simulink model "adc083000"  (R2013b)
settings: Solver=FixedStepDiscrete  SolverMode=SingleTasking  StartTime=0.0  StopTime=10.0  RelTol=1e-3
libraries: xbsIndex_r4 x18, xps_library x13, dspsigops x8
settings Model: Creator=franco  LastModifiedBy=root
settings DebuggingCC: SolverPrmCheckMsg=none  StateNameClashWarn=warning

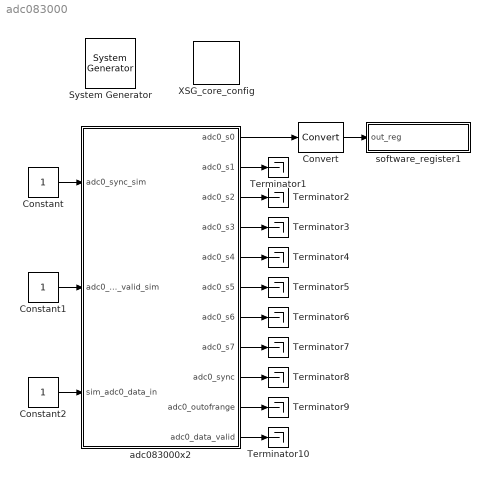
== system adc083000 ==
  " System Generator" : xbsIndex_r4/ System Generator  Tag=genX  xilinxfamily=virtex5  part=xc5vsx95t  speed=-1  package=ff1136  synthesis_tool=XST  clock_wrapper=Clock Enables  directory=./adc083000/sysgen  proj_type=Project Navigator  Synth_file=XST Defaults  Impl_file=ISE Defaults  testbench=off  simulink_period=1  sysclk_period=8.3333  dcm_input_clock_period=100  incr_netlist=off  trim_vbits=Everywhere in SubSystem  dbl_ovrd=According to Block Masks  core_generation=According to Block Masks  run_coregen=off  deprecated_control=off  eval_field=0  block_type=sysgen
  Constant : Constant
  Constant1 : Constant
  Constant2 : Constant
  Convert : xbsIndex_r4/Convert  gui_display_data_type=Fixed-point  arith_type=Unsigned  n_bits=32  bin_pt=0  float_type=Single  exp_bits=8  fraction_bits=24  quantization=Truncate  overflow=Wrap  en=off  latency=0  dbl_ovrd=off  pipeline=off  block_type=convert
  Terminator{1..10} (10 alike) : Terminator
  XSG_core_config : xps_library/XSG_core_config  Tag=xps:xsg  hw_sys=ROACH:sx95t  clk_src=adc0_clk  ROACH_clk_src=adc0_clk  ROACH2_clk_src=sys_clk  MKDIG_clk_src=sys_clk  clk_rate=120  sample_period=1  synthesis_tool=XST
  adc083000x2 : Subsystem  Tag=xps:adc083000x2  AncestorBlock=xps_library/adc083000x2  mask(adc_083000x2){use_adc0=on, use_adc1=off, demux_adc=off, clock_sync=off, verbose=off, using_ctrl=on, adc_clk_rate=480, sample_period=1, bit_width=8}
      mask prompts: use_adc0 "Use ZD0K0?"; use_adc1 "Use ZDOK1?"; demux_adc "Demux ADCs by 2?"; clock_sync "Interleave 2 ADC boards?"; verbose "Verbose Block Creation?"; using_ctrl "Add ports for control registers?"; adc_clk_rate "ADC clock rate (MHz)"; sample_period "Sample Period"; bit_width "Output Bit Width"
      mask help:
      | The ADC block converts analog inputs to digital outputs.
      | Every clock cycle, the inputs are sampled and digitized to
      | 8 bit binary point numbers in the range of [-1, 1).
      |
      | Online block-specific documentation: http://casper.berkeley.edu/wiki/Adc083000
      mask init:
      | adc083000_mask;
      mask Help: eval('xlWeb([getenv(''MLIB_ROOT''), ''\doc\html\sys_adc\sys_adc.html''])')
  software_register1 : Subsystem  Tag=xps:sw_reg  AncestorBlock=xps_library/software_register  mask(swreg){io_dir=To Processor, io_delay=0, sample_period=1, names=reg, bitwidths=32, bin_pts=0, arith_types=0, sim_port=off, show_format=on}
      mask prompts: io_dir "I/O direction"; io_delay "I/O delay"; sample_period "Sample period"; names "Bitfield names [msb...lsb]"; bitwidths "Bitfield widths"; bin_pts "Bitfield binary pts"; arith_types "Bitfield types, ufix=0, fix=1, bool=2"; sim_port "Provide sim input/output?"; show_format "Print format string?"
      mask help: A 32-bit software-accessible register. Can be divided into bitfields of varying widths and types using the fields in the block mask.
      mask init:
      | try
      |     swreg_init(gcb)
      | catch ex
      |     disp(sprintf('%s: %s', gcb, ex.message))
      |     errordlg(ex.message)
      | end
      settings: AttributesFormatString=1output:uf32.0 = 32 bits
      mask TypeOptions io_dir: To Processor | From Processor
      mask Callback io_dir:
      | mask_enables = get_param(gcb, 'MaskEnables');
      | mask_names = get_param(gcb, 'MaskNames');
      | if strcmp(get_param(gcb, 'io_dir'), 'To Processor'),
      |     mask_enables{ismember(mask_names, 'sample_period')} = 'off';
      | else
      |     mask_enables{ismember(mask_names, 'sample_period')} = 'on';
      | end
      | set_param(gcb, 'MaskEnables', mask_enables);
  wires:
  adc083000x2/1(adc0_s0) -> Convert/1
  adc083000x2/2(adc0_s1) -> Terminator1/1
  adc083000x2/3(adc0_s2) -> Terminator2/1
  adc083000x2/4(adc0_s3) -> Terminator3/1
  adc083000x2/5(adc0_s4) -> Terminator4/1
  adc083000x2/6(adc0_s5) -> Terminator5/1
  adc083000x2/7(adc0_s6) -> Terminator6/1
  adc083000x2/8(adc0_s7) -> Terminator7/1
  adc083000x2/9(adc0_sync) -> Terminator8/1
  adc083000x2/10(adc0_outofrange) -> Terminator9/1
  adc083000x2/11(adc0_data_valid) -> Terminator10/1
  Constant/1 -> adc083000x2/1(adc0_sync_sim)
  Constant1/1 -> adc083000x2/2(adc0_data_valid_sim)
  Constant2/1 -> adc083000x2/3(sim_adc0_data_in)
  Convert/1 -> software_register1/1(out_reg)

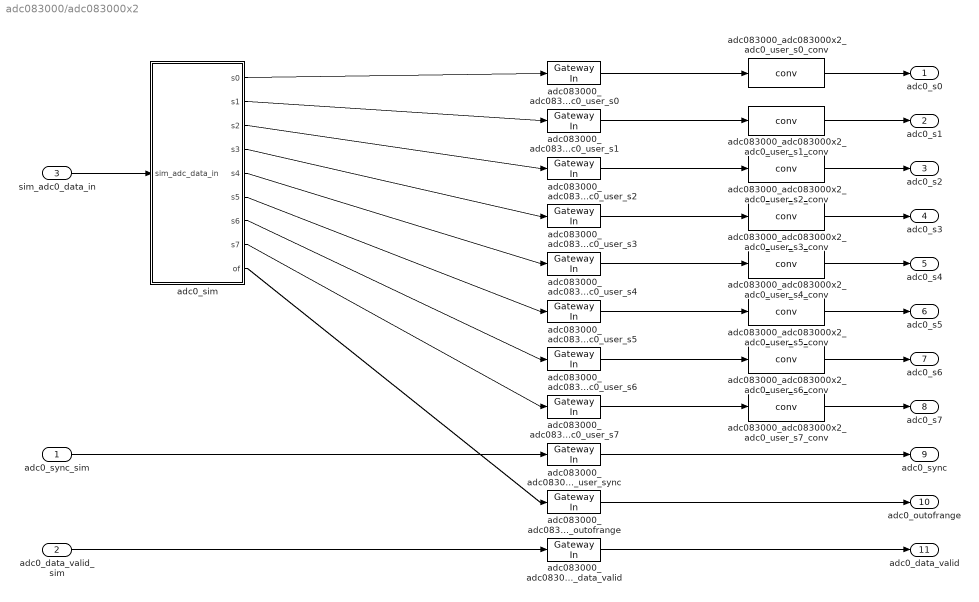
== system adc083000/adc083000x2 ==
  adc0_sync_sim : Inport
  adc0_data_valid_sim : Inport  Port=2
  sim_adc0_data_in : Inport  Port=3
  adc083000_adc083000x2_adc0_user_data_valid : xbsIndex_r4/Gateway In  gui_display_data_type=Fixed-point  arith_type=Unsigned  n_bits=1  bin_pt=0  preci_type=Single  exp_width=8  frac_width=24  quantization="Round  (unbiased: +/- Inf)"  overflow=Saturate  period=1  dbl_ovrd=off  timing_constraint=None  locs_specified=off  LOCs={}  UseAsADC=off  ADCChannel='1'  inherit_from_input=off  hdl_port=on  block_type=gatewayin
  adc083000_adc083000x2_adc0_user_outofrange : xbsIndex_r4/Gateway In  gui_display_data_type=Fixed-point  arith_type=Unsigned  n_bits=4  bin_pt=0  preci_type=Single  exp_width=8  frac_width=24  quantization="Round  (unbiased: +/- Inf)"  overflow=Saturate  period=1  dbl_ovrd=off  timing_constraint=None  locs_specified=off  LOCs={}  UseAsADC=off  ADCChannel='1'  inherit_from_input=off  hdl_port=on  block_type=gatewayin
  adc083000_adc083000x2_adc0_user_s{0..7} (8 alike) : xbsIndex_r4/Gateway In  gui_display_data_type=Fixed-point  arith_type=Unsigned  n_bits=8  bin_pt=0  preci_type=Single  exp_width=8  frac_width=24  quantization="Round  (unbiased: +/- Inf)"  overflow=Saturate  period=1  dbl_ovrd=off  timing_constraint=None  locs_specified=off  LOCs={}  UseAsADC=off  ADCChannel='1'  inherit_from_input=off  hdl_port=on  block_type=gatewayin
  adc083000_adc083000x2_adc0_user_s0_conv : xps_library/ADCs/conv  bit_width=8
  adc083000_adc083000x2_adc0_user_s1_conv : xps_library/ADCs/conv  bit_width=8
  adc083000_adc083000x2_adc0_user_s2_conv : xps_library/ADCs/conv  bit_width=8
  adc083000_adc083000x2_adc0_user_s3_conv : xps_library/ADCs/conv  bit_width=8
  adc083000_adc083000x2_adc0_user_s4_conv : xps_library/ADCs/conv  bit_width=8
  adc083000_adc083000x2_adc0_user_s5_conv : xps_library/ADCs/conv  bit_width=8
  adc083000_adc083000x2_adc0_user_s6_conv : xps_library/ADCs/conv  bit_width=8
  adc083000_adc083000x2_adc0_user_s7_conv : xps_library/ADCs/conv  bit_width=8
  adc083000_adc083000x2_adc0_user_sync : xbsIndex_r4/Gateway In  gui_display_data_type=Fixed-point  arith_type=Unsigned  n_bits=4  bin_pt=0  preci_type=Single  exp_width=8  frac_width=24  quantization="Round  (unbiased: +/- Inf)"  overflow=Saturate  period=1  dbl_ovrd=off  timing_constraint=None  locs_specified=off  LOCs={}  UseAsADC=off  ADCChannel='1'  inherit_from_input=off  hdl_port=on  block_type=gatewayin
  adc0_sim : Subsystem  AncestorBlock=xps_library/ADCs/adc_sim  mask(adc_sim){nStreams=8, bit_width=8}
      mask prompts: nStreams "Number of Output Streams"; bit_width "Sample Bit Width"
      mask help:
      | This block simulates the behavior of a demuxed ADC, which takes
      | as input a waveform and returns digital samples in parallel at
      | a slower rate.
      |
      | This block is used to simulate the behavior
      mask init:
      | adc_sim_init(gcb, ...
      |     'nStreams', nStreams, ...
      |     'bit_width', bit_width);
  adc0_s0 : Outport
  adc0_s1 : Outport  Port=2
  adc0_s2 : Outport  Port=3
  adc0_s3 : Outport  Port=4
  adc0_s4 : Outport  Port=5
  adc0_s5 : Outport  Port=6
  adc0_s6 : Outport  Port=7
  adc0_s7 : Outport  Port=8
  adc0_sync : Outport  Port=9
  adc0_outofrange : Outport  Port=10
  adc0_data_valid : Outport  Port=11
  wires:
  sim_adc0_data_in/1 -> adc0_sim/1(sim_adc_data_in)
  adc0_sim/1(s0) -> adc083000_adc083000x2_adc0_user_s0/1
  adc083000_adc083000x2_adc0_user_s0/1 -> adc083000_adc083000x2_adc0_user_s0_conv/1
  adc083000_adc083000x2_adc0_user_s0_conv/1 -> adc0_s0/1
  adc0_sim/2(s1) -> adc083000_adc083000x2_adc0_user_s1/1
  adc083000_adc083000x2_adc0_user_s1/1 -> adc083000_adc083000x2_adc0_user_s1_conv/1
  adc083000_adc083000x2_adc0_user_s1_conv/1 -> adc0_s1/1
  adc0_sim/3(s2) -> adc083000_adc083000x2_adc0_user_s2/1
  adc083000_adc083000x2_adc0_user_s2/1 -> adc083000_adc083000x2_adc0_user_s2_conv/1
  adc083000_adc083000x2_adc0_user_s2_conv/1 -> adc0_s2/1
  adc0_sim/4(s3) -> adc083000_adc083000x2_adc0_user_s3/1
  adc083000_adc083000x2_adc0_user_s3/1 -> adc083000_adc083000x2_adc0_user_s3_conv/1
  adc083000_adc083000x2_adc0_user_s3_conv/1 -> adc0_s3/1
  adc0_sim/5(s4) -> adc083000_adc083000x2_adc0_user_s4/1
  adc083000_adc083000x2_adc0_user_s4/1 -> adc083000_adc083000x2_adc0_user_s4_conv/1
  adc083000_adc083000x2_adc0_user_s4_conv/1 -> adc0_s4/1
  adc0_sim/6(s5) -> adc083000_adc083000x2_adc0_user_s5/1
  adc083000_adc083000x2_adc0_user_s5/1 -> adc083000_adc083000x2_adc0_user_s5_conv/1
  adc083000_adc083000x2_adc0_user_s5_conv/1 -> adc0_s5/1
  adc0_sim/7(s6) -> adc083000_adc083000x2_adc0_user_s6/1
  adc083000_adc083000x2_adc0_user_s6/1 -> adc083000_adc083000x2_adc0_user_s6_conv/1
  adc083000_adc083000x2_adc0_user_s6_conv/1 -> adc0_s6/1
  adc0_sim/8(s7) -> adc083000_adc083000x2_adc0_user_s7/1
  adc083000_adc083000x2_adc0_user_s7/1 -> adc083000_adc083000x2_adc0_user_s7_conv/1
  adc083000_adc083000x2_adc0_user_s7_conv/1 -> adc0_s7/1
  adc0_sync_sim/1 -> adc083000_adc083000x2_adc0_user_sync/1
  adc083000_adc083000x2_adc0_user_sync/1 -> adc0_sync/1
  adc0_sim/9(of) -> adc083000_adc083000x2_adc0_user_outofrange/1
  adc083000_adc083000x2_adc0_user_outofrange/1 -> adc0_outofrange/1
  adc0_data_valid_sim/1 -> adc083000_adc083000x2_adc0_user_data_valid/1
  adc083000_adc083000x2_adc0_user_data_valid/1 -> adc0_data_valid/1

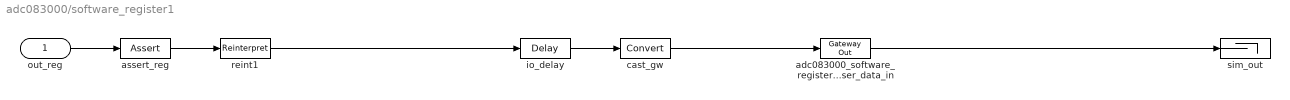
== system adc083000/software_register1 ==
  out_reg : Inport
  adc083000_software_register1_user_data_in : xbsIndex_r4/Gateway Out  inherit_from_input=off  hdl_port=on  timing_constraint=None  locs_specified=off  LOCs={}  UseAsDAC=off  DACChannel='1'  block_type=gatewayout
  assert_reg : xbsIndex_r4/Assert  assert_type=on  type_source=Explicitly  gui_display_data_type=Fixed-point  arith_type=Unsigned  n_bits=32  bin_pt=0  preci_type=Single  exp_width=8  frac_width=24  assert_rate=off  rate_source=Explicitly  period=1  output_port=on  block_type=assert
  cast_gw : xbsIndex_r4/Convert  gui_display_data_type=Fixed-point  arith_type=Unsigned  n_bits=32  bin_pt=0  float_type=Single  exp_bits=8  fraction_bits=24  quantization=Truncate  overflow=Wrap  en=off  latency=0  dbl_ovrd=off  pipeline=off  block_type=convert
  io_delay : xbsIndex_r4/Delay  rst=off  infoeditControl=Selection of Reset will increase slice count due to use of real FFs and instead of SRLs  en=off  latency=0  dbl_ovrd=off  reg_retiming=on  block_type=delay
  reint1 : xbsIndex_r4/Reinterpret  force_arith_type=on  arith_type=Unsigned  force_bin_pt=on  bin_pt=0  block_type=reinterpret
  sim_out : Terminator
  wires:
  io_delay/1 -> cast_gw/1
  cast_gw/1 -> adc083000_software_register1_user_data_in/1
  adc083000_software_register1_user_data_in/1 -> sim_out/1
  out_reg/1 -> assert_reg/1
  assert_reg/1 -> reint1/1
  reint1/1 -> io_delay/1

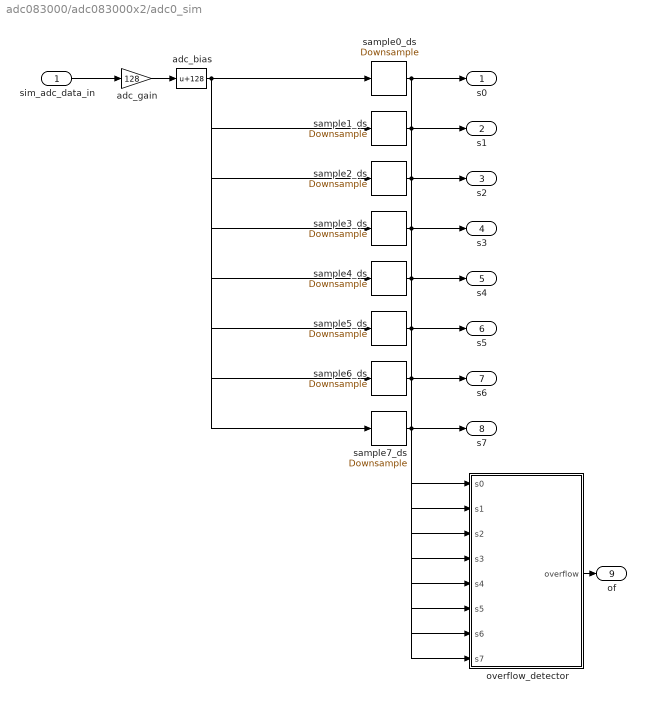
== system adc083000/adc083000x2/adc0_sim ==
  sim_adc_data_in : Inport
  adc_bias : Bias  Bias=128  SaturateOnIntegerOverflow=on
  adc_gain : Gain  Gain=128
  overflow_detector : Subsystem  AncestorBlock=xps_library/ADCs/of_detect_bus  mask(of_detect_bus){nStreams=8, bit_width=8}
      mask prompts: nStreams "Number of Streams"; bit_width "Bit Width"
      mask init:
      | of_detect_bus_init(gcb, ...
      |     'nStreams', nStreams, ...
      |     'bit_width', bit_width);
  sample0_ds : dspsigops/Downsample  N=8  phase=1  InputProcessing=Inherited (this choice will be removed - see release notes)  RateOptions=Enforce single-rate processing  smode=Force single rate  fmode=Maintain input frame rate  ic=0
  sample1_ds : dspsigops/Downsample  N=8  phase=2  InputProcessing=Inherited (this choice will be removed - see release notes)  RateOptions=Enforce single-rate processing  smode=Force single rate  fmode=Maintain input frame rate  ic=0
  sample2_ds : dspsigops/Downsample  N=8  phase=3  InputProcessing=Inherited (this choice will be removed - see release notes)  RateOptions=Enforce single-rate processing  smode=Force single rate  fmode=Maintain input frame rate  ic=0
  sample3_ds : dspsigops/Downsample  N=8  phase=4  InputProcessing=Inherited (this choice will be removed - see release notes)  RateOptions=Enforce single-rate processing  smode=Force single rate  fmode=Maintain input frame rate  ic=0
  sample4_ds : dspsigops/Downsample  N=8  phase=5  InputProcessing=Inherited (this choice will be removed - see release notes)  RateOptions=Enforce single-rate processing  smode=Force single rate  fmode=Maintain input frame rate  ic=0
  sample5_ds : dspsigops/Downsample  N=8  phase=6  InputProcessing=Inherited (this choice will be removed - see release notes)  RateOptions=Enforce single-rate processing  smode=Force single rate  fmode=Maintain input frame rate  ic=0
  sample6_ds : dspsigops/Downsample  N=8  phase=7  InputProcessing=Inherited (this choice will be removed - see release notes)  RateOptions=Enforce single-rate processing  smode=Force single rate  fmode=Maintain input frame rate  ic=0
  sample7_ds : dspsigops/Downsample  N=8  phase=0  InputProcessing=Inherited (this choice will be removed - see release notes)  RateOptions=Enforce single-rate processing  smode=Force single rate  fmode=Maintain input frame rate  ic=0
  s0 : Outport
  s1 : Outport  Port=2
  s2 : Outport  Port=3
  s3 : Outport  Port=4
  s4 : Outport  Port=5
  s5 : Outport  Port=6
  s6 : Outport  Port=7
  s7 : Outport  Port=8
  of : Outport  Port=9
  wires:
  sim_adc_data_in/1 -> adc_gain/1
  adc_gain/1 -> adc_bias/1
  overflow_detector/1(overflow) -> of/1
  adc_bias/1 -> sample0_ds/1, sample1_ds/1, sample2_ds/1, sample3_ds/1, sample4_ds/1, sample5_ds/1, sample6_ds/1, sample7_ds/1
  sample0_ds/1 -> overflow_detector/1(s0), s0/1
  sample1_ds/1 -> overflow_detector/2(s1), s1/1
  sample2_ds/1 -> overflow_detector/3(s2), s2/1
  sample3_ds/1 -> overflow_detector/4(s3), s3/1
  sample4_ds/1 -> overflow_detector/5(s4), s4/1
  sample5_ds/1 -> overflow_detector/6(s5), s5/1
  sample6_ds/1 -> overflow_detector/7(s6), s6/1
  sample7_ds/1 -> overflow_detector/8(s7), s7/1

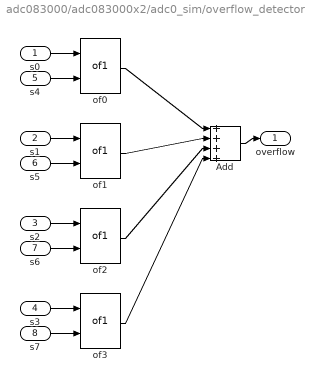
== system adc083000/adc083000x2/adc0_sim/overflow_detector ==
  s0 : Inport
  s1 : Inport  Port=2
  s2 : Inport  Port=3
  s3 : Inport  Port=4
  s4 : Inport  Port=5
  s5 : Inport  Port=6
  s6 : Inport  Port=7
  s7 : Inport  Port=8
  Add : Sum  Inputs=++++
  of{0..3} (4 alike) : xps_library/ADCs/of1  bit_num=0  n_adc_bits=8
  overflow : Outport
  wires:
  s0/1 -> of0/1
  s4/1 -> of0/2
  of0/1 -> Add/1
  s1/1 -> of1/1
  s5/1 -> of1/2
  of1/1 -> Add/2
  s2/1 -> of2/1
  s6/1 -> of2/2
  of2/1 -> Add/3
  s3/1 -> of3/1
  s7/1 -> of3/2
  of3/1 -> Add/4
  Add/1 -> overflow/1
